simulink model "Nonelinear_Control_Project"  (R2018b)
settings: Solver=VariableStepAuto  StartTime=0.0  StopTime=80  FixedStep=0.01  RelTol=1e-3
InitFcn:
  | Initial_Data
StopFcn:
  | Plots
values from neighbouring files (symbols this model uses):
  alpha1 = 10    [Initial_Data.m]
  alpha2 = 10    [Initial_Data.m]
  alpha3 = 10    [Initial_Data.m]
  alpha4 = 10    [Initial_Data.m]
  b = 5    [Initial_Data.m]
  beta1 = 1    [Initial_Data.m]
  beta2 = 1    [Initial_Data.m]
  beta3 = 1    [Initial_Data.m]
  beta4 = 1    [Initial_Data.m]
  c3 = 1    [Initial_Data.m]
  c4 = 6    [Initial_Data.m]
  c7 = 1    [Initial_Data.m]
  c8 = 6    [Initial_Data.m]
  cpsi = 1    [Initial_Data.m]
  cz = 1    [Initial_Data.m]
  eta1 = 2    [Initial_Data.m]
  eta2 = 2    [Initial_Data.m]
  g = 9.81    [Initial_Data.m]
  Ix = 0.022    [Initial_Data.m]
  Iy = 0.022    [Initial_Data.m]
  Iz = 0.042    [Initial_Data.m]
  Jr = 0    [Initial_Data.m]
  k1 = 0.001    [Initial_Data.m]
  k2 = 0.001    [Initial_Data.m]
  k3 = 0.001    [Initial_Data.m]
  k4 = 0.0012    [Initial_Data.m]
  k5 = 0.0012    [Initial_Data.m]
  k6 = 0.0012    [Initial_Data.m]
  l = 0.21    [Initial_Data.m]
  m = 1.1    [Initial_Data.m]
  m1 = 1    [Initial_Data.m]
  m2 = 1    [Initial_Data.m]
  mperim1 = 7    [Initial_Data.m]
  mperim2 = 7    [Initial_Data.m]
  mperim3 = 7    [Initial_Data.m]
  mperim4 = 7    [Initial_Data.m]
  n1 = 3    [Initial_Data.m]
  n2 = 3    [Initial_Data.m]
  nperim1 = 9    [Initial_Data.m]
  nperim2 = 9    [Initial_Data.m]
  nperim3 = 9    [Initial_Data.m]
  nperim4 = 9    [Initial_Data.m]
  omega = 2000    [Initial_Data.m]
  Phi_desired = 0    [Initial_Data.m]
  Phi_dot_desired = 0    [Initial_Data.m]
  Phi_doubledot_desired = 0    [Initial_Data.m]
  Psi_desired = 0.5    [Initial_Data.m]
  Psi_dot_desired = 0    [Initial_Data.m]
  Psi_doubledot_desired = 0    [Initial_Data.m]
  Psi_tiersdot_desired = 0    [Initial_Data.m]
  Teta_desired = 0    [Initial_Data.m]
  Teta_dot_desired = 0    [Initial_Data.m]
  Teta_doubledot_desired = 0    [Initial_Data.m]
  x_desired = 0.6    [Initial_Data.m]
  x_dot_desired = 0    [Initial_Data.m]
  x_doubledot_desired = 0    [Initial_Data.m]
  x_tiersdot_desired = 0    [Initial_Data.m]
  y_desired = 0.6    [Initial_Data.m]
  y_dot_desired = 0    [Initial_Data.m]
  y_doubledot_desired = 0    [Initial_Data.m]
  y_tiersdot_desired = 0    [Initial_Data.m]
  z_desired = 0.6    [Initial_Data.m]
  z_dot_desired = 0    [Initial_Data.m]
  z_doubledot_desired = 0    [Initial_Data.m]
  z_tiersdot_desired = 0    [Initial_Data.m]
undefined symbols (not defined in the file or in its folder): c, CD0, CDalpha, CDalphadot, CDdelE, CDiH, CDq, CDu, CL0, CLalpha, CLalphadot, Clbeta, Clbetadot, CldelA, CLdelE, CldelR, CLiH, Clp, CLq, Clr, ClT, CLu, Cm0, Cmalpha, Cmalphadot, CmdelE, cmiH, Cmq, CmT1, CmTalpha, CmTu, Cmu, Cnbeta, Cnbetadot, CndelA, CndelR, Cnp, Cnr, CnTbeta, CTxu, CTy, CTz, Cybeta, Cybetadot, CydelA, CydelR, Cyp, Cyr, delE, iH, Ixx, Ixz, Iyy, Izz, Kp, mass, Ro, S, T1, taw ... (+3)
libraries: simulink x1
(part 1 of 2)
settings Model: Creator=Mehdi RJ  LastModifiedBy=User
settings DataIOCC: LimitDataPoints=on  SaveFormat=Array  SignalLoggingSaveFormat=ModelDataLogs
settings OptimizationCC: BlockReduction=off  BooleanDataType=off  LifeSpan=inf
settings DebuggingCC: SaveWithParameterizedLinksMsg=none  UnderspecifiedInitializationDetection=Classic  MergeDetectMultiDrivingBlocksExec=none  SignalResolutionControl=TryResolveAllWithWarning  MultiTaskDSMMsg=warning  MultiTaskCondExecSysMsg=none  SFUnexpectedBacktrackingDiag=warning  SFNoUnconditionalDefaultTransitionDiag=warning  SFExecutionAtInitializationDiag=none
settings HardwareCC: ProdBitPerPointer=32  ProdBitPerSizeT=32  ProdBitPerPtrDiffT=32  ProdLargestAtomicFloat=None  ProdIntDivRoundTo=Undefined  ProdEndianess=Unspecified  ProdWordSize=32  ProdHWDeviceType=32-bit Generic  TargetUnknown=on
settings ModelReferenceCC: PropagateSignalLabelsOutOfModel=off
settings SFSimCC: SimUseLocalCustomCode=off
settings RTWCC: RTWUseLocalCustomCode=off
settings CodeAppCC: StateflowObjectComments=on
settings GRTTargetCC: TargetLangStandard=C89/C90 (ANSI)  GeneratePreprocessorConditionals=Disable all
settings ConfigComp: CovMetricSettings=dw  CovHtmlReporting=on  CovSaveCumulativeToWorkspaceVar=on  CovSaveSingleToWorkspaceVar=on  CovExternalEMLEnable=off

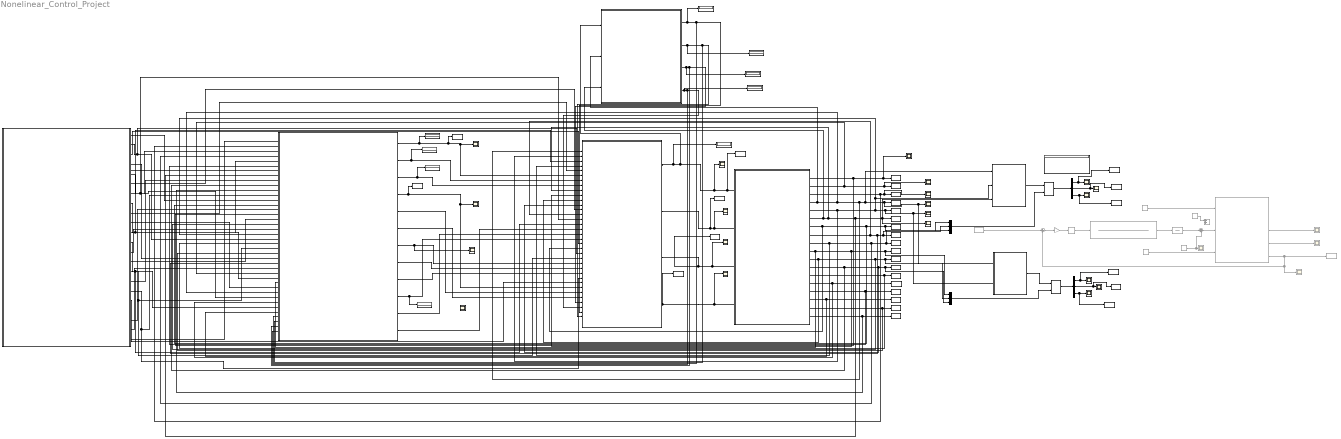
== system Nonelinear_Control_Project ==
  Add : Sum  Commented=on
  Airplane Dynamics : Subsystem  Commented=on
  "Controller " : Subsystem
  Demux : Demux  Outputs=3
  Demux2 : Demux  Outputs=3
  "Desired Values " : Subsystem
  Display{,1..9} (10 alike) : Display
  Gain1 : Gain  Commented=on  Gain=-1
  MATLAB Function : MATLAB Function  TreatAsAtomicUnit=on
  MATLAB Function1 : MATLAB Function  TreatAsAtomicUnit=on
  Matrix Multiply : Product  Multiplication=Matrix(*)
  Matrix Multiply1 : Product  Multiplication=Matrix(*)
  P : Scope
  PID Controller : simulink/Continuous/PID Controller  Commented=on  Controller=PID  Form=Parallel  TimeDomain=Continuous-time  SampleTime=-1  IntegratorMethod=Forward Euler  FilterMethod=Forward Euler  ControllerParametersSource=internal  P=9.72091586765638e-06  I=5.86209894111036e-08  D=9.64251086658951e-05  UseFilter=on  N=15.2377063472214  TunerSelectOption=Transfer Function Based (PID Tuner App)  InitialConditionSource=internal  InitialConditionForIntegrator=0  InitialConditionForFilter=0  DifferentiatorICPrevScaledInput=0  ExternalReset=none  TrackingMode=off  Kt=1  LimitOutput=off  UpperSaturationLimit=inf  LowerSaturationLimit=-inf  LinearizeAsGain=on  AntiWindupMode=none  Kb=1  POutMin=[]  POutMax=[]  IOutMin=[]  IOutMax=[]  DOutMin=[]  DOutMax=[]  NOutMin=[]  NOutMax=[]  SumOutMin=[]  SumOutMax=[]  SaturationOutMin=[]  SaturationOutMax=[]  PParamMin=[]  PParamMax=[]  IParamMin=[]  IParamMax=[]  DParamMin=[]  DParamMax=[]  NParamMin=[]  NParamMax=[]  KbParamMin=[]  KbParamMax=[]  KtParamMin=[]  KtParamMax=[]  KbOutMin=[]  KbOutMax=[]  KtOutMin=[]  KtOutMax=[]  IntegratorOutMin=[]  IntegratorOutMax=[]  FilterOutMin=[]  FilterOutMax=[]  SumI1OutMin=[]  SumI1OutMax=[]  SumI2OutMin=[]  SumI2OutMax=[]  SumI3OutMin=[]  SumI3OutMax=[]  SumI4OutMin=[]  SumI4OutMax=[]  SumDOutMin=[]  SumDOutMax=[]  DifferentiatorOutMin=[]  DifferentiatorOutMax=[]  FilterDiffOutCoefMin=[]  FilterDiffOutCoefMax=[]  ReciprocalOutMin=[]  ReciprocalOutMax=[]  SumDenOutMin=[]  SumDenOutMax=[]  SumNumOutMin=[]  SumNumOutMax=[]  DivideOutMin=[]  DivideOutMax=[]  IntegratorContinuousStateAttributes=''  IntegratorStateMustResolveToSignalObject=off  IntegratorRTWStateStorageClass=Auto  FilterContinuousStateAttributes=''  FilterStateMustResolveToSignalObject=off  FilterRTWStateStorageClass=Auto  ParallelPVariant=InternalParameters  IdealPVariant=Disabled  IVariant=InternalParameters  DVariant=InternalParameters  IntegratorVariant=Continuous  SatVariant=Disabled  AWVariant=Passthrough  PCopyVariant=Disabled  TRVariant=Disabled  FdbkBlocksVariant=Forward  IdealPFdbkVariant=Disabled  SatFdbkVariant=Disabled  DerivativeFilterVariant=ContFilter  NVariant=InternalParameters  NCopyVariant=Disabled  FilterICVariant=InternalICsFilter  IntegratorICVariant=InternalICs  ExternalResetVariant=Disabled  TRSumVariant=Passthrough  SumFdbkVariant=Disabled  SumVariant=Sum_PID
  Pilot Transfer Function : TransferFcn  Commented=on  Numerator=[(- Kp*TL* taw) (- Kp*taw+ 2*Kp*TL) (2*Kp)]  Denominator=[(TI*TN*taw) (TN*taw+TI*taw+2*TI*TN) (taw+2*TN+2*TI) 2]
  Pulse Generator : DiscretePulseGenerator  Commented=on  PulseType=Time based  Amplitude=0.0175*5  Period=2000  PhaseDelay=800
  Q : Scope
  Quadrotordynamics : Subsystem
  R : Scope
  Scope{,1..3} (4 alike) : Scope  Commented=on
  Scope{4..17} (14 alike) : Scope
  Subsystem : Subsystem
  Sum : Sum  Commented=on  Inputs=|+-
  Sum1 : Sum  Commented=on  Inputs=|++
  TSMC and SMC Manifolds : Subsystem
  To Workspace : ToWorkspace  VariableName=x  SaveFormat=Timeseries  SampleTime=-1
  To Workspace1 : ToWorkspace  VariableName=y  SaveFormat=Timeseries  SampleTime=-1
  To Workspace10 : ToWorkspace  VariableName=Tetadot  SaveFormat=Timeseries  SampleTime=-1
  To Workspace11 : ToWorkspace  VariableName=Psidot  SaveFormat=Timeseries  SampleTime=-1
  To Workspace12 : ToWorkspace  VariableName=xddot  SaveFormat=Timeseries  SampleTime=-1
  To Workspace13 : ToWorkspace  VariableName=yddot  SaveFormat=Timeseries  SampleTime=-1
  To Workspace14 : ToWorkspace  VariableName=zddot  SaveFormat=Timeseries  SampleTime=-1
  To Workspace15 : ToWorkspace  VariableName=Phiddot  SaveFormat=Timeseries  SampleTime=-1
  To Workspace16 : ToWorkspace  VariableName=Tetaddot  SaveFormat=Timeseries  SampleTime=-1
  To Workspace17 : ToWorkspace  VariableName=Psiddot  SaveFormat=Timeseries  SampleTime=-1
  To Workspace18 : ToWorkspace  VariableName=P  SaveFormat=Timeseries  SampleTime=-1
  To Workspace19 : ToWorkspace  VariableName=Q  SaveFormat=Timeseries  SampleTime=-1
  To Workspace2 : ToWorkspace  VariableName=z  SaveFormat=Timeseries  SampleTime=-1
  To Workspace20 : ToWorkspace  Commented=on  VariableName=h  SaveFormat=Timeseries  SampleTime=-1
  To Workspace21 : ToWorkspace  VariableName=R  SaveFormat=Timeseries  SampleTime=-1
  To Workspace22 : ToWorkspace  VariableName=U  SaveFormat=Timeseries  SampleTime=-1
  To Workspace23 : ToWorkspace  VariableName=V  SaveFormat=Timeseries  SampleTime=-1
  To Workspace24 : ToWorkspace  VariableName=W  SaveFormat=Timeseries  SampleTime=-1
  To Workspace25 : ToWorkspace  VariableName=u1  SaveFormat=Timeseries  SampleTime=-1
  To Workspace26 : ToWorkspace  VariableName=u2  SaveFormat=Timeseries  SampleTime=-1
  To Workspace27 : ToWorkspace  VariableName=u3  SaveFormat=Timeseries  SampleTime=-1
  To Workspace28 : ToWorkspace  VariableName=u4  SaveFormat=Timeseries  SampleTime=-1
  To Workspace29 : ToWorkspace  VariableName=s1  SaveFormat=Timeseries  SampleTime=-1
  To Workspace3 : ToWorkspace  VariableName=Phi  SaveFormat=Timeseries  SampleTime=-1
  To Workspace30 : ToWorkspace  VariableName=s3  SaveFormat=Timeseries  SampleTime=-1
  To Workspace4 : ToWorkspace  VariableName=Teta  SaveFormat=Timeseries  SampleTime=-1
  To Workspace5 : ToWorkspace  VariableName=Psi  SaveFormat=Timeseries  SampleTime=-1
  To Workspace6 : ToWorkspace  VariableName=xdot  SaveFormat=Timeseries  SampleTime=-1
  To Workspace7 : ToWorkspace  VariableName=ydot  SaveFormat=Timeseries  SampleTime=-1
  To Workspace8 : ToWorkspace  VariableName=zdot  SaveFormat=Timeseries  SampleTime=-1
  To Workspace9 : ToWorkspace  VariableName=Phidot  SaveFormat=Timeseries  SampleTime=-1
  Transfer Fcn1 : TransferFcn  Commented=on  Numerator=[10]  Denominator=[1 10]
  U : Scope
  V : Scope
  Vector Concatenate : Concatenate  NumInputs=3
  Vector Concatenate1 : Concatenate  NumInputs=3
  W : Scope
  delA : Constant  Commented=on  Value=0
  delA1 : Constant  Commented=on  Value=delE
  delR : Constant  Commented=on  Value=0
  h : Constant  Commented=on  Value=20000
  wires:
  delR/1 -> Airplane Dynamics/3(delR)
  delA/1 -> Airplane Dynamics/1(delA)
  Airplane Dynamics/3(Theta) -> Scope/1
  h/1 -> Sum/1
  Airplane Dynamics/4(Q) -> Scope1/1
  Pulse Generator/1 -> Sum1/2, Scope2/1
  Sum/1 -> Gain1/1
  Gain1/1 -> PID Controller/1
  Airplane Dynamics/5(h) -> Sum/2, Scope3/1, To Workspace20/1
  Pilot Transfer Function/1 -> Transfer Fcn1/1
  Transfer Fcn1/1 -> Sum1/1
  PID Controller/1 -> Pilot Transfer Function/1
  delA1/1 -> Add/1
  Sum1/1 -> Airplane Dynamics/2(delE)
  Quadrotordynamics/1(x) -> TSMC and SMC Manifolds/16(x), Scope4/1, To Workspace/1
  Quadrotordynamics/2(y) -> TSMC and SMC Manifolds/28(y), Scope5/1, To Workspace1/1
  Quadrotordynamics/3(z) -> TSMC and SMC Manifolds/2(z), Scope6/1, To Workspace2/1
  Quadrotordynamics/4(Phi) -> Subsystem/2(Phi), TSMC and SMC Manifolds/32(Phi), To Workspace3/1, MATLAB Function1/1(Phi), Scope7/1, MATLAB Function/1(Phi), "Controller "/1(Phi)
  "Controller "/1(u1) -> Display7/1, Subsystem/1(u1), Scope10/1, To Workspace25/1, Quadrotordynamics/1(u1)
  "Controller "/2(u2) -> To Workspace26/1, Scope11/1, Quadrotordynamics/2(u2)
  "Controller "/3(u3) -> Scope12/1, Quadrotordynamics/3(u3), To Workspace27/1
  "Controller "/4(u4) -> Scope13/1, Quadrotordynamics/4(u4), To Workspace28/1
  Quadrotordynamics/7(xdot) -> "Controller "/21(xdot), TSMC and SMC Manifolds/14(xdot), Vector Concatenate/1, To Workspace6/1
  Quadrotordynamics/5(Teta) -> "Controller "/2(Teta), TSMC and SMC Manifolds/20(Teta), MATLAB Function/2(Teta), MATLAB Function1/2(Teta), Scope8/1, To Workspace4/1
  Quadrotordynamics/10(Phidot) -> TSMC and SMC Manifolds/30(Phidot), "Controller "/10(Phidot), Vector Concatenate1/1, To Workspace9/1
  Quadrotordynamics/11(Tetadot) -> "Controller "/11(Tetadot), TSMC and SMC Manifolds/18(Tetadot), Vector Concatenate1/2, To Workspace10/1
  Quadrotordynamics/8(ydot) -> "Controller "/14(ydot), TSMC and SMC Manifolds/26(ydot), Vector Concatenate/2, To Workspace7/1
  TSMC and SMC Manifolds/1("s1 ") -> Display/1, To Workspace29/1, "Controller "/6(s1), Scope14/1
  TSMC and SMC Manifolds/2("s1dot ") -> Display8/1, "Controller "/7(s1dot)
  TSMC and SMC Manifolds/3("s2 ") -> Display1/1, "Controller "/8(s2)
  TSMC and SMC Manifolds/4("s3 ") -> To Workspace30/1, Scope15/1, "Controller "/29(s3)
  TSMC and SMC Manifolds/5("s3dot ") -> "Controller "/30(s3dot)
  TSMC and SMC Manifolds/6("s4 ") -> "Controller "/31(s4)
  TSMC and SMC Manifolds/7("s5 ") -> Scope16/1, "Controller "/24(s5)
  TSMC and SMC Manifolds/8("s5dot  ") -> "Controller "/25(s5dot)
  TSMC and SMC Manifolds/9("s6 ") -> "Controller "/26(s6)
  TSMC and SMC Manifolds/10("s7 ") -> Display2/1, "Controller "/19(s7)
  TSMC and SMC Manifolds/11("s7dot ") -> "Controller "/18(s7dot)
  TSMC and SMC Manifolds/12("s8 ") -> "Controller "/17(s8)
  Quadrotordynamics/6(Psi) -> Subsystem/3(Psi), Scope9/1, To Workspace5/1, MATLAB Function/3(Psi), TSMC and SMC Manifolds/8(Psi), "Controller "/9(Psi)
  Quadrotordynamics/12(Psidot) -> "Controller "/12(Psidot), Vector Concatenate1/3, To Workspace11/1, TSMC and SMC Manifolds/10(Psidot)
  Quadrotordynamics/15(zddot) -> TSMC and SMC Manifolds/6(zdoubledot), To Workspace14/1
  Quadrotordynamics/13(xddot) -> TSMC and SMC Manifolds/22(xdoubledot), To Workspace12/1
  Quadrotordynamics/14(yddot) -> TSMC and SMC Manifolds/34(ydoubledot), To Workspace13/1
  Quadrotordynamics/17(Tetaddot) -> TSMC and SMC Manifolds/24(Tetadoubledot), To Workspace16/1
  Quadrotordynamics/18(Psiddot) -> TSMC and SMC Manifolds/11(Psidoubledot), To Workspace17/1
  Quadrotordynamics/16(Phiddot) -> To Workspace15/1, TSMC and SMC Manifolds/36(Phidoubledot)
  "Desired Values "/7("z_dot_desired ") -> TSMC and SMC Manifolds/3(z_dot_desired)
  "Desired Values "/16("Psi_dot_desired ") -> TSMC and SMC Manifolds/9(Psi_dot_desired)
  "Desired Values "/17("Psi_doubledot_desired ") -> "Controller "/27(Psi_doubledot_desired), TSMC and SMC Manifolds/12(Psi_doubledot_desired)
  "Desired Values "/1("x_dot_desired ") -> TSMC and SMC Manifolds/13(x_dot_desired)
  "Desired Values "/2("x_doubledot_desired ") -> "Controller "/22(x_doubledot_desired), TSMC and SMC Manifolds/21(x_doubledot_desired)
  "Desired Values "/4("y_dot_desired ") -> TSMC and SMC Manifolds/25(y_dot_desired)
  "Desired Values "/5("y_doubledot_desired ") -> "Controller "/15(y_doubledot_desired), TSMC and SMC Manifolds/33(y_doubledot_desired)
  "Desired Values "/10("Phi_desired ") -> TSMC and SMC Manifolds/31(Phi_desired)
  "Desired Values "/11("Phi_dot_desired ") -> TSMC and SMC Manifolds/29(Phi_dot_desired)
  "Desired Values "/12("Phi_doubledot_desired ") -> "Controller "/16(Phi_doubledot_desired), TSMC and SMC Manifolds/35(Phi_doubledot_desired)
  "Desired Values "/13("Teta_desired ") -> TSMC and SMC Manifolds/19(Teta_desired)
  "Desired Values "/14("Teta_dot_desired  ") -> TSMC and SMC Manifolds/17(Teta_dot_desired)
  "Desired Values "/15("Teta_doubledot_desired ") -> "Controller "/23(Teta_doubledot_desired), TSMC and SMC Manifolds/23(Teta_doubledot_desired)
  "Desired Values "/8("z_doubledot_desired ") -> "Controller "/3(z_doubledot_desired), TSMC and SMC Manifolds/5(z_doubledot_desired)
  "Desired Values "/9("z_tiersdot_desired ") -> "Controller "/5(z_tiersdot_desired)
  "Desired Values "/6("y_tiersdot_desired ") -> "Controller "/13(y_tiersdot_desired)
  "Desired Values "/3("x_tiersdot_desired ") -> "Controller "/20(x_tiersdot_desired)
  "Desired Values "/18("Psi_tiersdot_desired ") -> "Controller "/28(Psi_tiersdot_desired)
  Subsystem/1("c1 ") -> Display3/1, TSMC and SMC Manifolds/37(c1), "Controller "/34(c1)
  Subsystem/3("c5 ") -> Display5/1, TSMC and SMC Manifolds/39(c5), "Controller "/32(c5)
  Subsystem/4("c6 ") -> Display6/1, TSMC and SMC Manifolds/40(c6), "Controller "/33(c6)
  Subsystem/2("c2 ") -> Display4/1, TSMC and SMC Manifolds/38(c2), "Controller "/35(c2)
  MATLAB Function/1(DCM) -> Matrix Multiply/1
  Quadrotordynamics/9(zdot) -> "Controller "/4(zdot), TSMC and SMC Manifolds/4("zdot "), Vector Concatenate/3, To Workspace8/1
  Vector Concatenate/1 -> Matrix Multiply/2
  Matrix Multiply/1 -> Demux/1
  Demux/3 -> To Workspace24/1, W/1
  Demux/2 -> To Workspace23/1, V/1
  Demux/1 -> To Workspace22/1, U/1
  MATLAB Function1/1(DCM) -> Matrix Multiply1/1
  Vector Concatenate1/1 -> Matrix Multiply1/2
  Demux2/1 -> To Workspace18/1, P/1
  Demux2/2 -> To Workspace19/1, Q/1
  Demux2/3 -> To Workspace21/1, R/1
  Matrix Multiply1/1 -> Demux2/1
  "Desired Values "/19("Psi_desired ") -> TSMC and SMC Manifolds/7("Psi_desired ")
  "Desired Values "/20("x_desired ") -> TSMC and SMC Manifolds/15(x_desired)
  "Desired Values "/21("y_desired ") -> TSMC and SMC Manifolds/27(y_desired)
  "Desired Values "/22("z_desired ") -> TSMC and SMC Manifolds/1("z_desired ")

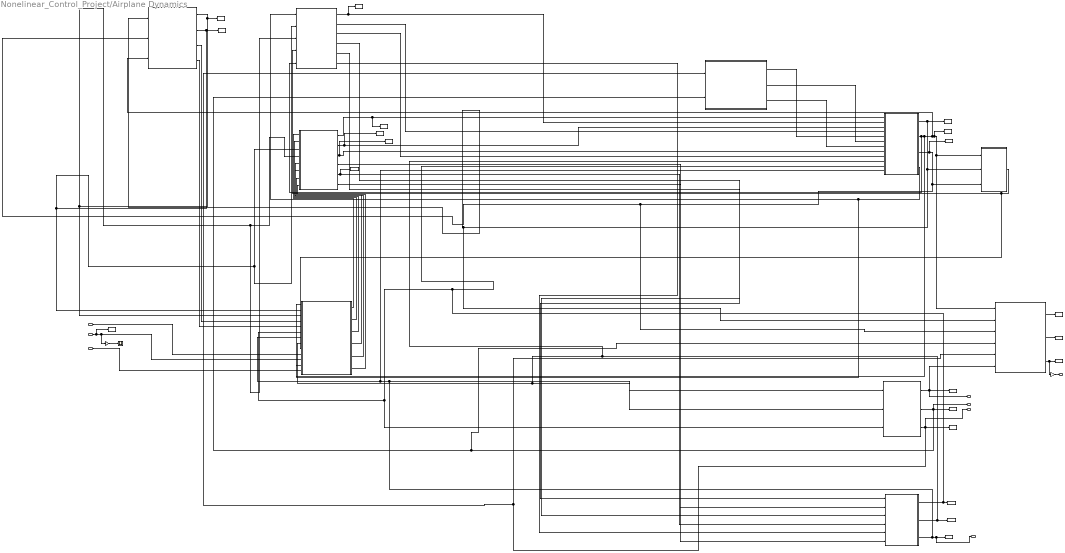
== system Nonelinear_Control_Project/Airplane Dynamics ==
  delA : Inport
  delE : Inport  Port=2
  delR : Inport  Port=3
  AnglesBlock : Subsystem
  Angular Velocities (P,Q,R) : Subsystem
  Body Aerodynamic Forces and Moments (FAxB,FAyB,FAzB,LAB,MAB,NAB) : Subsystem
  Dynamic Pressure : Subsystem
  Euler's Angles (Phi,Theta,Psi) : Subsystem
  GBlock : Subsystem
  Gain : Gain  Gain=-1
  Gain1 : Gain  Gain=180/pi
  Linear Velocities (U,V,W) : Subsystem
  Navigation : Subsystem
  Scope : Scope
  Stability Aerodunamic Forces and Moments (FAxS,FAyS,FAzS,LAS,MAS,NAS) : Subsystem
  Thrust Forces and Moments (FTx,FTy,FTz,LT,MT,NT) : Subsystem
  To Workspace : ToWorkspace  VariableName=XInertia  SaveFormat=Timeseries  SampleTime=-1
  To Workspace1 : ToWorkspace  VariableName=YInertia  SaveFormat=Timeseries  SampleTime=-1
  To Workspace10 : ToWorkspace  VariableName=Q  SaveFormat=Timeseries  SampleTime=-1
  To Workspace11 : ToWorkspace  VariableName=R  SaveFormat=Timeseries  SampleTime=-1
  To Workspace12 : ToWorkspace  VariableName=P  SaveFormat=Timeseries  SampleTime=-1
  To Workspace13 : ToWorkspace  VariableName=W  SaveFormat=Timeseries  SampleTime=-1
  To Workspace14 : ToWorkspace  VariableName=FAzB  SaveFormat=Timeseries  SampleTime=-1
  To Workspace15 : ToWorkspace  VariableName=FTx  SaveFormat=Timeseries  SampleTime=-1
  To Workspace16 : ToWorkspace  VariableName=FAxB  SaveFormat=Timeseries  SampleTime=-1
  To Workspace17 : ToWorkspace  VariableName=FAyB  SaveFormat=Timeseries  SampleTime=-1
  To Workspace18 : ToWorkspace  VariableName=V  SaveFormat=Timeseries  SampleTime=-1
  To Workspace19 : ToWorkspace  VariableName=delE  SaveFormat=Timeseries  SampleTime=-1
  To Workspace2 : ToWorkspace  VariableName=ZInertia  SaveFormat=Timeseries  SampleTime=-1
  To Workspace3 : ToWorkspace  VariableName=alpha  SaveFormat=Timeseries  SampleTime=-1
  To Workspace4 : ToWorkspace  VariableName=beta  SaveFormat=Timeseries  SampleTime=-1
  To Workspace5 : ToWorkspace  VariableName=U  SaveFormat=Timeseries  SampleTime=-1
  To Workspace6 : ToWorkspace  VariableName=Psi  SaveFormat=Timeseries  SampleTime=-1
  To Workspace7 : ToWorkspace  VariableName=Phi  SaveFormat=Timeseries  SampleTime=-1
  To Workspace8 : ToWorkspace  VariableName=Theta  SaveFormat=Timeseries  SampleTime=-1
  To Workspace9 : ToWorkspace  VariableName=MAB  SaveFormat=Timeseries  SampleTime=-1
  Psi : Outport
  Phi : Outport  Port=2
  Theta : Outport  Port=3
  Q : Outport  Port=4
  h : Outport  Port=5
  wires:
  AnglesBlock/2(alpha) -> To Workspace3/1, Thrust Forces and Moments (FTx,FTy,FTz,LT,MT,NT)/2(alpha), Body Aerodynamic Forces and Moments (FAxB,FAyB,FAzB,LAB,MAB,NAB)/3(alpha), Stability Aerodunamic Forces and Moments (FAxS,FAyS,FAzS,LAS,MAS,NAS)/2(alpha)
  Stability Aerodunamic Forces and Moments (FAxS,FAyS,FAzS,LAS,MAS,NAS)/1(FAxS) -> Body Aerodynamic Forces and Moments (FAxB,FAyB,FAzB,LAB,MAB,NAB)/1(FAxS)
  Thrust Forces and Moments (FTx,FTy,FTz,LT,MT,NT)/2(FTy) -> Linear Velocities (U,V,W)/4(FTy)
  Thrust Forces and Moments (FTx,FTy,FTz,LT,MT,NT)/5(MT) -> Angular Velocities (P,Q,R)/3(MT)
  Angular Velocities (P,Q,R)/1(P) -> To Workspace12/1, Linear Velocities (U,V,W)/11(P), Stability Aerodunamic Forces and Moments (FAxS,FAyS,FAzS,LAS,MAS,NAS)/6(P), Euler's Angles (Phi,Theta,Psi)/3(P)
  AnglesBlock/3(betadot) -> Stability Aerodunamic Forces and Moments (FAxS,FAyS,FAzS,LAS,MAS,NAS)/4("betadot ")
  Euler's Angles (Phi,Theta,Psi)/1(Psi) -> To Workspace6/1, Navigation/6(Psi), Psi/1
  delR/1 -> Stability Aerodunamic Forces and Moments (FAxS,FAyS,FAzS,LAS,MAS,NAS)/13(delR)
  Body Aerodynamic Forces and Moments (FAxB,FAyB,FAzB,LAB,MAB,NAB)/4(LAB) -> Angular Velocities (P,Q,R)/2(LAB)
  Body Aerodynamic Forces and Moments (FAxB,FAyB,FAzB,LAB,MAB,NAB)/5(MAB) -> To Workspace9/1, Angular Velocities (P,Q,R)/4(MAB)
  Linear Velocities (U,V,W)/3(W) -> To Workspace13/1, Dynamic Pressure/3(W), AnglesBlock/2(W), Navigation/3(W)
  Angular Velocities (P,Q,R)/3(Q) -> Euler's Angles (Phi,Theta,Psi)/2(Q), Linear Velocities (U,V,W)/12(Q), Stability Aerodunamic Forces and Moments (FAxS,FAyS,FAzS,LAS,MAS,NAS)/7(Q), Q/1, To Workspace10/1
  Linear Velocities (U,V,W)/1(V) -> To Workspace18/1, Dynamic Pressure/2(V), AnglesBlock/1(V), Navigation/2(V)
  Euler's Angles (Phi,Theta,Psi)/3(Theta) -> To Workspace8/1, GBlock/1(Theta), Navigation/5(Theta), Theta/1
  AnglesBlock/1("beta ") -> To Workspace4/1, Body Aerodynamic Forces and Moments (FAxB,FAyB,FAzB,LAB,MAB,NAB)/4(beta), Thrust Forces and Moments (FTx,FTy,FTz,LT,MT,NT)/3(beta), Stability Aerodunamic Forces and Moments (FAxS,FAyS,FAzS,LAS,MAS,NAS)/3(beta)
  Linear Velocities (U,V,W)/4(delU) -> Stability Aerodunamic Forces and Moments (FAxS,FAyS,FAzS,LAS,MAS,NAS)/1(delU), Thrust Forces and Moments (FTx,FTy,FTz,LT,MT,NT)/1(delU)
  Thrust Forces and Moments (FTx,FTy,FTz,LT,MT,NT)/3(FTz) -> Linear Velocities (U,V,W)/9(FTz)
  Navigation/2(YInertia) -> To Workspace1/1
  Stability Aerodunamic Forces and Moments (FAxS,FAyS,FAzS,LAS,MAS,NAS)/4(LAS) -> Body Aerodynamic Forces and Moments (FAxB,FAyB,FAzB,LAB,MAB,NAB)/6(LAS)
  Euler's Angles (Phi,Theta,Psi)/2(Phi) -> To Workspace7/1, Navigation/4(Phi), GBlock/2("Phi "), Phi/1
  Body Aerodynamic Forces and Moments (FAxB,FAyB,FAzB,LAB,MAB,NAB)/3(FAzB) -> To Workspace14/1, Linear Velocities (U,V,W)/8(FAzB)
  Stability Aerodunamic Forces and Moments (FAxS,FAyS,FAzS,LAS,MAS,NAS)/2(FAyS) -> Body Aerodynamic Forces and Moments (FAxB,FAyB,FAzB,LAB,MAB,NAB)/2(FAyS)
  GBlock/2(gy) -> Linear Velocities (U,V,W)/6(gy)
  AnglesBlock/4(alphadot) -> Stability Aerodunamic Forces and Moments (FAxS,FAyS,FAzS,LAS,MAS,NAS)/5(alphadot)
  Navigation/1(XInertia) -> To Workspace/1
  Thrust Forces and Moments (FTx,FTy,FTz,LT,MT,NT)/1(FTx) -> To Workspace15/1, Linear Velocities (U,V,W)/2(FTx)
  Stability Aerodunamic Forces and Moments (FAxS,FAyS,FAzS,LAS,MAS,NAS)/5(MAS) -> Body Aerodynamic Forces and Moments (FAxB,FAyB,FAzB,LAB,MAB,NAB)/7(MAS)
  Thrust Forces and Moments (FTx,FTy,FTz,LT,MT,NT)/6(NT) -> Angular Velocities (P,Q,R)/5(NT)
  Stability Aerodunamic Forces and Moments (FAxS,FAyS,FAzS,LAS,MAS,NAS)/6(NAS) -> Body Aerodynamic Forces and Moments (FAxB,FAyB,FAzB,LAB,MAB,NAB)/8(NAS)
  Navigation/3(ZInertia) -> Gain/1, To Workspace2/1
  Linear Velocities (U,V,W)/2(U) -> Thrust Forces and Moments (FTx,FTy,FTz,LT,MT,NT)/5(U), Stability Aerodunamic Forces and Moments (FAxS,FAyS,FAzS,LAS,MAS,NAS)/12(U), AnglesBlock/3(U), To Workspace5/1, Navigation/1(U), Dynamic Pressure/1(U)
  Stability Aerodunamic Forces and Moments (FAxS,FAyS,FAzS,LAS,MAS,NAS)/3(FAzS) -> Body Aerodynamic Forces and Moments (FAxB,FAyB,FAzB,LAB,MAB,NAB)/5(FAzS)
  Dynamic Pressure/1(q1) -> Stability Aerodunamic Forces and Moments (FAxS,FAyS,FAzS,LAS,MAS,NAS)/9(q1), Thrust Forces and Moments (FTx,FTy,FTz,LT,MT,NT)/4(q1)
  Body Aerodynamic Forces and Moments (FAxB,FAyB,FAzB,LAB,MAB,NAB)/6(NAB) -> Angular Velocities (P,Q,R)/6(NAB)
  GBlock/1(gx) -> Linear Velocities (U,V,W)/5(gx)
  GBlock/3(gz) -> Linear Velocities (U,V,W)/7(gz)
  Body Aerodynamic Forces and Moments (FAxB,FAyB,FAzB,LAB,MAB,NAB)/1(FAxB) -> To Workspace16/1, Linear Velocities (U,V,W)/1(FAxB)
  Angular Velocities (P,Q,R)/2(R) -> To Workspace11/1, Stability Aerodunamic Forces and Moments (FAxS,FAyS,FAzS,LAS,MAS,NAS)/8(R), Euler's Angles (Phi,Theta,Psi)/1(R), Linear Velocities (U,V,W)/10(R)
  Thrust Forces and Moments (FTx,FTy,FTz,LT,MT,NT)/4(LT) -> Angular Velocities (P,Q,R)/1(LT)
  Body Aerodynamic Forces and Moments (FAxB,FAyB,FAzB,LAB,MAB,NAB)/2(FAyB) -> To Workspace17/1, Linear Velocities (U,V,W)/3(FAyB)
  delA/1 -> Stability Aerodunamic Forces and Moments (FAxS,FAyS,FAzS,LAS,MAS,NAS)/10(delA)
  Gain/1 -> h/1
  delE/1 -> To Workspace19/1, Gain1/1, Stability Aerodunamic Forces and Moments (FAxS,FAyS,FAzS,LAS,MAS,NAS)/11(delE)
  Gain1/1 -> Scope/1

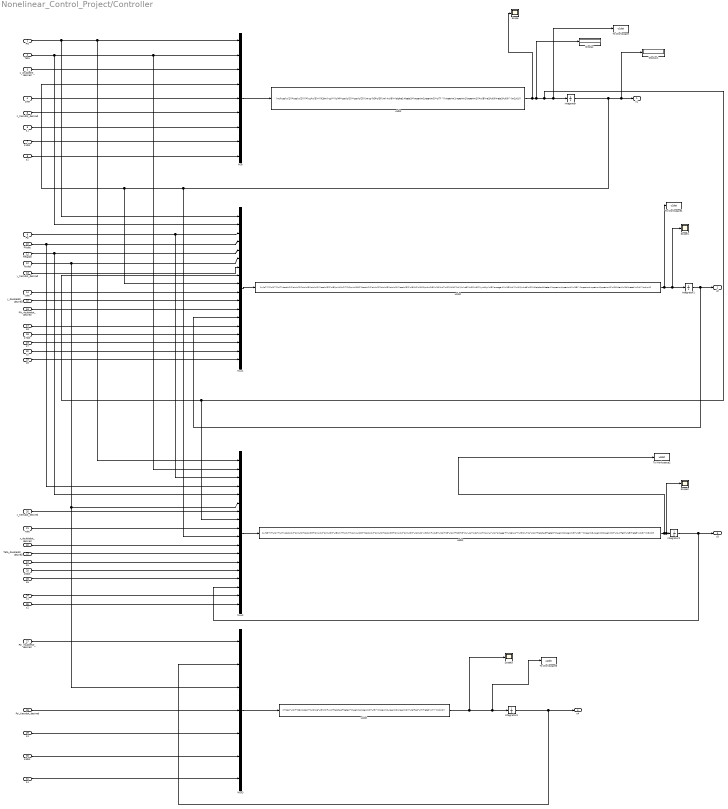
== system Nonelinear_Control_Project/Controller  ==
  Phi : Inport
  Teta : Inport  Port=2
  z_doubledot_desired : Inport  Port=3
  zdot : Inport  Port=4
  z_tiersdot_desired : Inport  Port=5
  s1 : Inport  Port=6
  s1dot : Inport  Port=7
  s2 : Inport  Port=8
  Psi : Inport  Port=9
  Phidot : Inport  Port=10
  Tetadot : Inport  Port=11
  Psidot : Inport  Port=12
  y_tiersdot_desired : Inport  Port=13
  ydot : Inport  Port=14
  y_doubledot_desired : Inport  Port=15
  Phi_doubledot_desired : Inport  Port=16
  s8 : Inport  Port=17
  s7dot : Inport  Port=18
  s7 : Inport  Port=19
  x_tiersdot_desired : Inport  Port=20
  xdot : Inport  Port=21
  x_doubledot_desired : Inport  Port=22
  Teta_doubledot_desired : Inport  Port=23
  s5 : Inport  Port=24
  s5dot : Inport  Port=25
  s6 : Inport  Port=26
  Psi_doubledot_desired : Inport  Port=27
  Psi_tiersdot_desired : Inport  Port=28
  s3 : Inport  Port=29
  s3dot : Inport  Port=30
  s4 : Inport  Port=31
  c5 : Inport  Port=32
  c6 : Inport  Port=33
  c1 : Inport  Port=34
  c2 : Inport  Port=35
  Display : Display
  Display1 : Display
  Integrator : Integrator  InitialCondition=0.0000001
  Integrator1 : Integrator
  Integrator2 : Integrator
  Integrator3 : Integrator
  Mux : Mux  Inputs=9
  Mux1 : Mux  Inputs=18
  Mux2 : Mux  Inputs=18
  Mux3 : Mux  Inputs=7
  Scope{,1..3} (4 alike) : Scope
  To Workspace : ToWorkspace  VariableName=u1dot  SaveFormat=Timeseries  SampleTime=-1
  To Workspace1 : ToWorkspace  VariableName=u2dot  SaveFormat=Timeseries  SampleTime=-1
  To Workspace2 : ToWorkspace  VariableName=u3dot  SaveFormat=Timeseries  SampleTime=-1
  To Workspace3 : ToWorkspace  VariableName=u4dot  SaveFormat=Timeseries  SampleTime=-1
  u1dot : Fcn  Expr=(m/(cos(u(1))*cos(u(2))))*(cz*u(3)+((k3/m)-cz)*((u(4)*cos(u(1))*cos(u(2)))/m-g-(k3*u(5))/m)+u(6)+(alpha1+beta1*(mperim1/nperim1)*u(7)^((mperim1-nperim1)/nperim1))*u(8)+e1*u(9)+eta1*u(9)^(m1/n1))
  u2dot : Fcn  Expr=(Ix/(c7*l))*(u(17)*(u(7)-(cos(u(1))*sin(u(2))*sin(u(3))-sin(u(1))*cos(u(3)))*u(8)/m)+((u(17)*k2/m)-u(18))*((cos(u(1))*sin(u(2))*sin(u(3))-sin(u(1))*cos(u(3)))*u(9)-k2*u(10))/m+u(18)*u(11)+c7*u(12)+((c7*k4*l/Ix)-c8)*(u(5)*u(6)*(Iy-Iz)+Jr*u(5)*omega+l*u(13)-k4*l*u(4))/Ix+c8*u(12)+(alpha4+beta4*(mperim4/nperim4)*u(16)^((mperim4-nperim4)/nperim4))*u(15)+e4*u(14)+eta4*u(14)^(m4/n4))
  u3dot : Fcn  Expr=(Iy/(c3*l))*(u(17)*(u(7)-(cos(u(1))*sin(u(2))*cos(u(3))+sin(u(1))*sin(u(3)))*u(8)/m)+((u(17)*k1/m)-u(18))*((cos(u(1))*sin(u(2))*cos(u(3))+sin(u(1))*sin(u(3)))*u(10)-k1*u(9))/m+u(18)*u(11)+c3*u(12)+((c3*k5*l/Iy)-c4)*(u(6)*u(4)*(Iz-Ix)-Jr*u(4)*omega+l*u(16)-k4*l*u(5))/Iy+c4*u(12)+(alpha3+beta3*(mperim3/nperim3)*u(13)^((mperim3-nperim3)/nperim3))*u(14)+e3*u(15)+eta3*u(15)^(m3/n3))
  u4dot : Fcn  Expr=Iz*(cpsi*u(1)+((k6/Iz)-cpsi)*((u(2)-k6*u(3))/Iz)+u(4)+(alpha2+beta2*(mperim2/nperim2)*u(5)^((mperim2-nperim2)/nperim2))*u(6)+e2*u(7)+eta2*u(7)^(m2/n2))
  u1 : Outport
  u2 : Outport  Port=2
  u3 : Outport  Port=3
  u4 : Outport  Port=4
  wires:
  z_doubledot_desired/1 -> Mux/3
  u1dot/1 -> Scope/1, Display/1, Mux2/8, Mux1/8, To Workspace/1, Integrator/1
  zdot/1 -> Mux/5
  z_tiersdot_desired/1 -> Mux/6
  s1/1 -> Mux/7
  s1dot/1 -> Mux/8
  s2/1 -> Mux/9
  Mux1/1 -> u2dot/1
  u2dot/1 -> To Workspace1/1, Scope1/1, Integrator1/1
  Psi/1 -> Mux2/3, Mux1/3
  Phidot/1 -> Mux2/4, Mux1/4
  Tetadot/1 -> Mux2/5, Mux1/5
  y_tiersdot_desired/1 -> Mux1/7
  ydot/1 -> Mux1/10
  y_doubledot_desired/1 -> Mux1/11
  Phi_doubledot_desired/1 -> Mux1/12
  s8/1 -> Mux1/14
  s7dot/1 -> Mux1/15
  s7/1 -> Mux1/16
  Integrator2/1 -> u3/1, Mux2/16
  u3dot/1 -> To Workspace2/1, Scope2/1, Integrator2/1
  Mux2/1 -> u3dot/1
  Phi/1 -> Mux2/1, Mux/1, Mux1/1
  Teta/1 -> Mux2/2, Mux/2, Mux1/2
  x_tiersdot_desired/1 -> Mux2/7
  xdot/1 -> Mux2/9
  Integrator/1 -> Mux2/10, Mux1/9, Mux/4, Display1/1, u1/1
  x_doubledot_desired/1 -> Mux2/11
  Teta_doubledot_desired/1 -> Mux2/12
  s5/1 -> Mux2/13
  s5dot/1 -> Mux2/14
  s6/1 -> Mux2/15
  Mux3/1 -> u4dot/1
  u4dot/1 -> Scope3/1, To Workspace3/1, Integrator3/1
  Integrator3/1 -> u4/1, Mux3/2
  Psi_doubledot_desired/1 -> Mux3/1
  Psidot/1 -> Mux3/3, Mux2/6, Mux1/6
  Psi_tiersdot_desired/1 -> Mux3/4
  s4/1 -> Mux3/7
  s3/1 -> Mux3/5
  s3dot/1 -> Mux3/6
  Integrator1/1 -> Mux1/13, u2/1
  c5/1 -> Mux1/17
  c6/1 -> Mux1/18
  c1/1 -> Mux2/17
  c2/1 -> Mux2/18
  Mux/1 -> u1dot/1

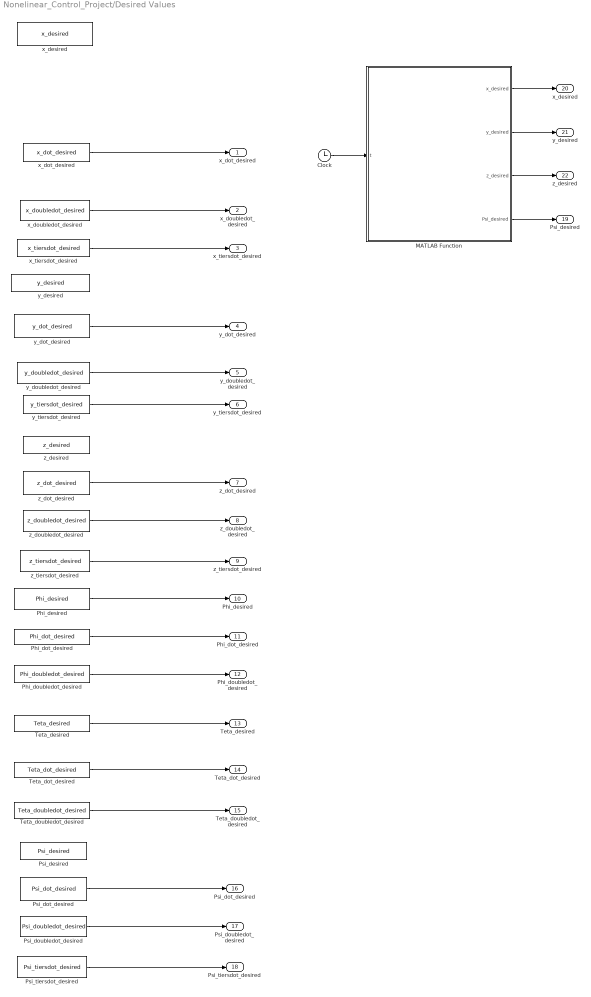
== system Nonelinear_Control_Project/Desired Values  ==
  Clock : Clock
  MATLAB Function : MATLAB Function  TreatAsAtomicUnit=on
  Phi_desired : Constant  Value=Phi_desired
  Phi_dot_desired : Constant  Value=Phi_dot_desired
  Phi_doubledot_desired : Constant  Value=Phi_doubledot_desired
  Psi_desired : Constant  Value=Psi_desired
  Psi_dot_desired : Constant  Value=Psi_dot_desired
  Psi_doubledot_desired : Constant  Value=Psi_doubledot_desired
  Psi_tiersdot_desired : Constant  Value=Psi_tiersdot_desired
  Teta_desired : Constant  Value=Teta_desired
  Teta_dot_desired : Constant  Value=Teta_dot_desired
  Teta_doubledot_desired : Constant  Value=Teta_doubledot_desired
  x_desired : Constant  Value=x_desired
  x_dot_desired : Constant  Value=x_dot_desired
  x_doubledot_desired : Constant  Value=x_doubledot_desired
  x_tiersdot_desired : Constant  Value=x_tiersdot_desired
  y_desired : Constant  Value=y_desired
  y_dot_desired : Constant  Value=y_dot_desired
  y_doubledot_desired : Constant  Value=y_doubledot_desired
  y_tiersdot_desired : Constant  Value=y_tiersdot_desired
  z_desired : Constant  Value=z_desired
  z_dot_desired : Constant  Value=z_dot_desired
  z_doubledot_desired : Constant  Value=z_doubledot_desired
  z_tiersdot_desired : Constant  Value=z_tiersdot_desired
  "x_dot_desired " : Outport
  "x_doubledot_desired " : Outport  Port=2
  "x_tiersdot_desired " : Outport  Port=3
  "y_dot_desired " : Outport  Port=4
  "y_doubledot_desired " : Outport  Port=5
  "y_tiersdot_desired " : Outport  Port=6
  "z_dot_desired " : Outport  Port=7
  "z_doubledot_desired " : Outport  Port=8
  "z_tiersdot_desired " : Outport  Port=9
  "Phi_desired " : Outport  Port=10
  "Phi_dot_desired " : Outport  Port=11
  "Phi_doubledot_desired " : Outport  Port=12
  "Teta_desired " : Outport  Port=13
  "Teta_dot_desired  " : Outport  Port=14
  "Teta_doubledot_desired " : Outport  Port=15
  "Psi_dot_desired " : Outport  Port=16
  "Psi_doubledot_desired " : Outport  Port=17
  "Psi_tiersdot_desired " : Outport  Port=18
  "Psi_desired " : Outport  Port=19
  "x_desired " : Outport  Port=20
  "y_desired " : Outport  Port=21
  "z_desired " : Outport  Port=22
  wires:
  y_dot_desired/1 -> "y_dot_desired "/1
  z_tiersdot_desired/1 -> "z_tiersdot_desired "/1
  x_doubledot_desired/1 -> "x_doubledot_desired "/1
  Teta_dot_desired/1 -> "Teta_dot_desired  "/1
  x_tiersdot_desired/1 -> "x_tiersdot_desired "/1
  z_dot_desired/1 -> "z_dot_desired "/1
  y_doubledot_desired/1 -> "y_doubledot_desired "/1
  Teta_doubledot_desired/1 -> "Teta_doubledot_desired "/1
  z_doubledot_desired/1 -> "z_doubledot_desired "/1
  Teta_desired/1 -> "Teta_desired "/1
  Phi_desired/1 -> "Phi_desired "/1
  y_tiersdot_desired/1 -> "y_tiersdot_desired "/1
  x_dot_desired/1 -> "x_dot_desired "/1
  Phi_doubledot_desired/1 -> "Phi_doubledot_desired "/1
  Phi_dot_desired/1 -> "Phi_dot_desired "/1
  Psi_tiersdot_desired/1 -> "Psi_tiersdot_desired "/1
  Psi_dot_desired/1 -> "Psi_dot_desired "/1
  Psi_doubledot_desired/1 -> "Psi_doubledot_desired "/1
  Clock/1 -> MATLAB Function/1(t)
  MATLAB Function/4(Psi_desired) -> "Psi_desired "/1
  MATLAB Function/1(x_desired) -> "x_desired "/1
  MATLAB Function/2(y_desired) -> "y_desired "/1
  MATLAB Function/3(z_desired) -> "z_desired "/1

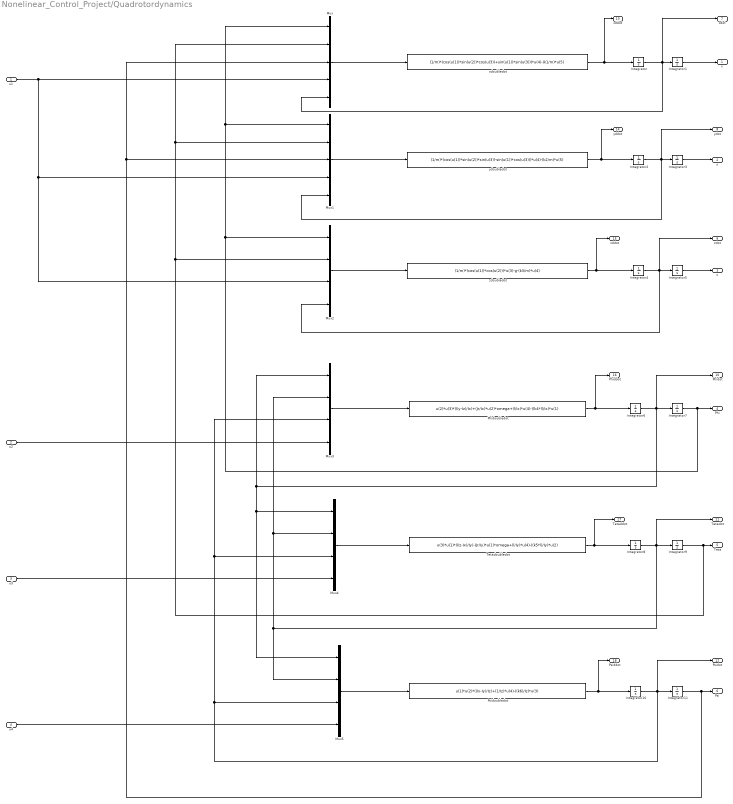
== system Nonelinear_Control_Project/Quadrotordynamics ==
  u1 : Inport
  u2 : Inport  Port=2
  u3 : Inport  Port=3
  u4 : Inport  Port=4
  Integrator{,1..11} (12 alike) : Integrator
  Mux : Mux  Inputs=5
  Mux1 : Mux  Inputs=5
  Mux{2..5} (4 alike) : Mux
  Phidoubledot : Fcn  Expr=u(2)*u(3)*((Iy-Iz)/Ix)+(Jr/Ix)*u(2)*omega+(l/Ix)*u(4)-((k4*l)/Ix)*u(1)
  Psidoubledot : Fcn  Expr=u(1)*u(2)*((Ix-Iy)/Iz)+(1/Iz)*u(4)-((k6)/Iz)*u(3)
  Tetadoubledot : Fcn  Expr=u(3)*u(1)*((Iz-Ix)/Iy)-(Jr/Iy)*u(1)*omega+(l/Iy)*u(4)-((k5*l)/Iy)*u(2)
  xdoubledot : Fcn  Expr=(1/m)*(cos(u(1))*sin(u(2))*cos(u(3))+sin(u(1))*sin(u(3)))*u(4)-(k1/m)*u(5)
  ydoubledot : Fcn  Expr=(1/m)*(cos(u(1))*sin(u(2))*sin(u(3))-sin(u(1))*cos(u(3)))*u(4)-(k2/m)*u(5)
  zdoubledot : Fcn  Expr=(1/m)*(cos(u(1))*cos(u(2)))*u(3)-g-(k3/m)*u(4)
  x : Outport
  y : Outport  Port=2
  z : Outport  Port=3
  Phi : Outport  Port=4
  Teta : Outport  Port=5
  Psi : Outport  Port=6
  xdot : Outport  Port=7
  ydot : Outport  Port=8
  zdot : Outport  Port=9
  Phidot : Outport  Port=10
  Tetadot : Outport  Port=11
  Psidot : Outport  Port=12
  xddot : Outport  Port=13
  yddot : Outport  Port=14
  zddot : Outport  Port=15
  Phiddot : Outport  Port=16
  Tetaddot : Outport  Port=17
  Psiddot : Outport  Port=18
  wires:
  ydoubledot/1 -> yddot/1, Integrator2/1
  Psidoubledot/1 -> Psiddot/1, Integrator10/1
  Integrator10/1 -> Psidot/1, Mux5/3, Mux4/3, Mux3/3, Integrator11/1
  Integrator6/1 -> Phidot/1, Mux5/1, Mux4/1, Mux3/1, Integrator7/1
  Phidoubledot/1 -> Phiddot/1, Integrator6/1
  Tetadoubledot/1 -> Tetaddot/1, Integrator8/1
  Integrator8/1 -> Tetadot/1, Mux5/2, Mux4/2, Mux3/2, Integrator9/1
  Integrator7/1 -> Mux/1, Mux1/1, Mux2/1, Phi/1
  xdoubledot/1 -> xddot/1, Integrator/1
  Integrator2/1 -> Mux1/5, ydot/1, Integrator3/1
  zdoubledot/1 -> zddot/1, Integrator4/1
  Integrator3/1 -> y/1
  Integrator4/1 -> Integrator5/1, zdot/1, Mux2/4
  Integrator/1 -> xdot/1, Mux/5, Integrator1/1
  Integrator9/1 -> Mux2/2, Mux1/2, Mux/2, Teta/1
  Integrator1/1 -> x/1
  Integrator5/1 -> z/1
  Integrator11/1 -> Mux1/3, Mux/3, Psi/1
  Mux/1 -> xdoubledot/1
  Mux1/1 -> ydoubledot/1
  Mux2/1 -> zdoubledot/1
  u1/1 -> Mux/4, Mux1/4, Mux2/3
  u2/1 -> Mux3/4
  u4/1 -> Mux5/4
  u3/1 -> Mux4/4
  Mux3/1 -> Phidoubledot/1
  Mux4/1 -> Tetadoubledot/1
  Mux5/1 -> Psidoubledot/1

== system Nonelinear_Control_Project/Subsystem ==
  u1 : Inport
  Phi : Inport  Port=2
  Psi : Inport  Port=3
  Mux : Mux  Inputs=3
  Mux1 : Mux  Inputs=2
  c1 : Fcn  Expr=(12*m)/(u(1)*cos(u(2))*cos(u(3)))
  c2 : Fcn  Expr=(8*m)/(u(1)*cos(u(2))*cos(u(3)))
  c5 : Fcn  Expr=(-12*m)/(u(1)*cos(u(2)))
  c6 : Fcn  Expr=(-8*m)/(u(1)*cos(u(2)))
  "c1 " : Outport
  "c2 " : Outport  Port=2
  "c5 " : Outport  Port=3
  "c6 " : Outport  Port=4
  wires:
  c5/1 -> "c5 "/1
  c1/1 -> "c1 "/1
  c2/1 -> "c2 "/1
  c6/1 -> "c6 "/1
  u1/1 -> Mux/1, Mux1/1
  Phi/1 -> Mux/2
  Psi/1 -> Mux/3, Mux1/2
  Mux/1 -> c2/1, c1/1
  Mux1/1 -> c5/1, c6/1

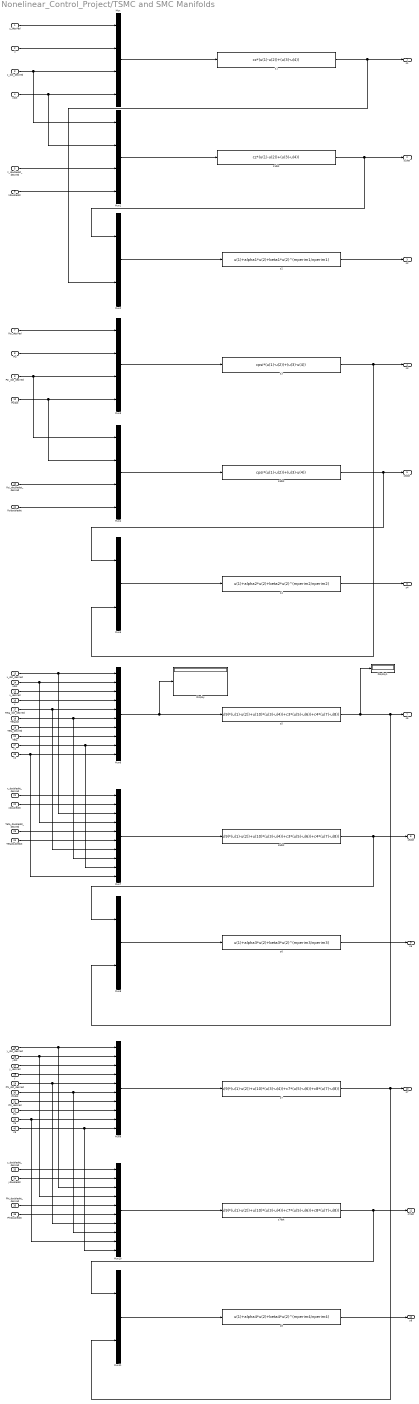
== system Nonelinear_Control_Project/TSMC and SMC Manifolds ==
  "z_desired " : Inport
  z : Inport  Port=2
  z_dot_desired : Inport  Port=3
  "zdot " : Inport  Port=4
  z_doubledot_desired : Inport  Port=5
  zdoubledot : Inport  Port=6
  "Psi_desired " : Inport  Port=7
  Psi : Inport  Port=8
  Psi_dot_desired : Inport  Port=9
  Psidot : Inport  Port=10
  Psidoubledot : Inport  Port=11
  Psi_doubledot_desired : Inport  Port=12
  x_dot_desired : Inport  Port=13
  xdot : Inport  Port=14
  x_desired : Inport  Port=15
  x : Inport  Port=16
  Teta_dot_desired : Inport  Port=17
  Tetadot : Inport  Port=18
  Teta_desired : Inport  Port=19
  Teta : Inport  Port=20
  x_doubledot_desired : Inport  Port=21
  xdoubledot : Inport  Port=22
  Teta_doubledot_desired : Inport  Port=23
  Tetadoubledot : Inport  Port=24
  y_dot_desired : Inport  Port=25
  ydot : Inport  Port=26
  y_desired : Inport  Port=27
  y : Inport  Port=28
  Phi_dot_desired : Inport  Port=29
  Phidot : Inport  Port=30
  Phi_desired : Inport  Port=31
  Phi : Inport  Port=32
  y_doubledot_desired : Inport  Port=33
  ydoubledot : Inport  Port=34
  Phi_doubledot_desired : Inport  Port=35
  Phidoubledot : Inport  Port=36
  c1 : Inport  Port=37
  c2 : Inport  Port=38
  c5 : Inport  Port=39
  c6 : Inport  Port=40
  Display : Display
  Display1 : Display
  Mux{,1,3..4} (4 alike) : Mux
  Mux{6..7,9..10} (4 alike) : Mux  Inputs=10
  Mux{2,5,8,11} (4 alike) : Mux  Inputs=2
  s1 : Fcn  Expr=cz*(u(1)-u(2))+(u(3)-u(4))
  s1dot : Fcn  Expr=cz*(u(1)-u(2))+(u(3)-u(4))
  s2 : Fcn  Expr=u(1)+alpha1*u(2)+beta1*u(2)^(mperim1/nperim1)
  s3 : Fcn  Expr=cpsi*(u(1)-u(2))+(u(3)-u(4))
  s3dot : Fcn  Expr=cpsi*(u(1)-u(2))+(u(3)-u(4))
  s4 : Fcn  Expr=u(1)+alpha2*u(2)+beta2*u(2)^(mperim2/nperim2)
  s5 : Fcn  Expr=u(9)*(u(1)-u(2))+u(10)*(u(3)-u(4))+c3*(u(5)-u(6))+c4*(u(7)-u(8))
  s5dot : Fcn  Expr=u(9)*(u(1)-u(2))+u(10)*(u(3)-u(4))+c3*(u(5)-u(6))+c4*(u(7)-u(8))
  s6 : Fcn  Expr=u(1)+alpha3*u(2)+beta3*u(2)^(mperim3/nperim3)
  s7 : Fcn  Expr=u(9)*(u(1)-u(2))+u(10)*(u(3)-u(4))+c7*(u(5)-u(6))+c8*(u(7)-u(8))
  s7dot : Fcn  Expr=u(9)*(u(1)-u(2))+u(10)*(u(3)-u(4))+c7*(u(5)-u(6))+c8*(u(7)-u(8))
  s8 : Fcn  Expr=u(1)+alpha4*u(2)+beta4*u(2)^(mperim4/nperim4)
  "s1 " : Outport
  "s1dot " : Outport  Port=2
  "s2 " : Outport  Port=3
  "s3 " : Outport  Port=4
  "s3dot " : Outport  Port=5
  "s4 " : Outport  Port=6
  "s5 " : Outport  Port=7
  "s5dot  " : Outport  Port=8
  "s6 " : Outport  Port=9
  "s7 " : Outport  Port=10
  "s7dot " : Outport  Port=11
  "s8 " : Outport  Port=12
  wires:
  Mux/1 -> s1/1
  "z_desired "/1 -> Mux/1
  z/1 -> Mux/2
  z_dot_desired/1 -> Mux/3, Mux1/1
  "zdot "/1 -> Mux/4, Mux1/2
  Mux1/1 -> s1dot/1
  zdoubledot/1 -> Mux1/4
  z_doubledot_desired/1 -> Mux1/3
  Mux2/1 -> s2/1
  s1/1 -> Mux2/2, "s1 "/1
  s1dot/1 -> Mux2/1, "s1dot "/1
  s2/1 -> "s2 "/1
  s3/1 -> Mux5/2, "s3 "/1
  Mux3/1 -> s3/1
  Mux4/1 -> s3dot/1
  s3dot/1 -> Mux5/1, "s3dot "/1
  Psidoubledot/1 -> Mux4/4
  Psi_dot_desired/1 -> Mux4/1, Mux3/3
  Psidot/1 -> Mux4/2, Mux3/4
  Psi/1 -> Mux3/2
  "Psi_desired "/1 -> Mux3/1
  Psi_doubledot_desired/1 -> Mux4/3
  s4/1 -> "s4 "/1
  Mux5/1 -> s4/1
  Mux6/1 -> Display/1, s5/1
  s5/1 -> Display1/1, Mux8/2, "s5 "/1
  x_dot_desired/1 -> Mux6/1, Mux7/3
  xdot/1 -> Mux7/4, Mux6/2
  x_desired/1 -> Mux6/3
  x/1 -> Mux6/4
  Teta_dot_desired/1 -> Mux7/7, Mux6/5
  Tetadot/1 -> Mux7/8, Mux6/6
  Teta_desired/1 -> Mux6/7
  Teta/1 -> Mux6/8
  s5dot/1 -> Mux8/1, "s5dot  "/1
  Mux7/1 -> s5dot/1
  x_doubledot_desired/1 -> Mux7/1
  xdoubledot/1 -> Mux7/2
  Teta_doubledot_desired/1 -> Mux7/5
  Tetadoubledot/1 -> Mux7/6
  s6/1 -> "s6 "/1
  Mux8/1 -> s6/1
  Phidoubledot/1 -> Mux10/6
  y_dot_desired/1 -> Mux9/1, Mux10/3
  ydoubledot/1 -> Mux10/2
  s7/1 -> Mux11/2, "s7 "/1
  Mux9/1 -> s7/1
  s8/1 -> "s8 "/1
  y_desired/1 -> Mux9/3
  Phi_doubledot_desired/1 -> Mux10/5
  y_doubledot_desired/1 -> Mux10/1
  Phi/1 -> Mux9/8
  Phi_desired/1 -> Mux9/7
  Mux10/1 -> s7dot/1
  ydot/1 -> Mux10/4, Mux9/2
  y/1 -> Mux9/4
  Phi_dot_desired/1 -> Mux10/7, Mux9/5
  s7dot/1 -> Mux11/1, "s7dot "/1
  Phidot/1 -> Mux10/8, Mux9/6
  Mux11/1 -> s8/1
  c1/1 -> Mux6/9, Mux7/9
  c2/1 -> Mux6/10, Mux7/10
  c5/1 -> Mux9/9, Mux10/9
  c6/1 -> Mux9/10, Mux10/10

== system Nonelinear_Control_Project/Airplane Dynamics/AnglesBlock ==
  V : Inport
  W : Inport  Port=2
  U : Inport  Port=3
  Atan2 : Trigonometry  Operator=atan2
  Derivative : Derivative
  Derivative1 : Derivative
  Divide : Product  Inputs=*/
  Scope : Scope
  Sin : Trigonometry  Operator=asin
  "beta " : Outport
  alpha : Outport  Port=2
  betadot : Outport  Port=3
  alphadot : Outport  Port=4
  wires:
  U/1 -> Atan2/2, Divide/2
  W/1 -> Atan2/1
  V/1 -> Divide/1
  Atan2/1 -> Derivative1/1, Scope/1, alpha/1
  Sin/1 -> Derivative/1, "beta "/1
  Divide/1 -> Sin/1
  Derivative/1 -> betadot/1
  Derivative1/1 -> alphadot/1

== system Nonelinear_Control_Project/Airplane Dynamics/Angular Velocities (P,Q,R) ==
  LT : Inport
  LAB : Inport  Port=2
  MT : Inport  Port=3
  MAB : Inport  Port=4
  NT : Inport  Port=5
  NAB : Inport  Port=6
  PBlock : Subsystem
  QBlock : Subsystem
  RBlock : Subsystem
  Scope : Scope
  P : Outport
  R : Outport  Port=2
  Q : Outport  Port=3
  wires:
  PBlock/2(Pdot) -> RBlock/3(Pdot)
  PBlock/1(P) -> RBlock/5(P), QBlock/3(P), P/1
  RBlock/2("Rdot ") -> PBlock/3(Rdot)
  LT/1 -> PBlock/2(LT)
  MAB/1 -> QBlock/1(MAB)
  LAB/1 -> PBlock/1(LAB)
  RBlock/1(R) -> R/1, PBlock/4(R), QBlock/4(R)
  NAB/1 -> RBlock/1(NAB)
  NT/1 -> RBlock/2(NT)
  MT/1 -> QBlock/2(MT)
  QBlock/1(Q) -> PBlock/5(Q), RBlock/4(Q), Scope/1, Q/1

== system Nonelinear_Control_Project/Airplane Dynamics/Body Aerodynamic Forces and Moments (FAxB,FAyB,FAzB,LAB,MAB,NAB) ==
  FAxS : Inport
  FAyS : Inport  Port=2
  alpha : Inport  Port=3
  beta : Inport  Port=4
  FAzS : Inport  Port=5
  LAS : Inport  Port=6
  MAS : Inport  Port=7
  NAS : Inport  Port=8
  FAxBBlock : Subsystem
  FAyBBlock : Subsystem
  FAzBBlock : Subsystem
  LABBlock : Subsystem
  MABBlock : Subsystem
  NABBlock : Subsystem
  FAxB : Outport
  FAyB : Outport  Port=2
  FAzB : Outport  Port=3
  LAB : Outport  Port=4
  MAB : Outport  Port=5
  NAB : Outport  Port=6
  wires:
  LAS/1 -> NABBlock/1(LAS), MABBlock/1(LAS), LABBlock/1(LAS)
  NAS/1 -> NABBlock/3(NAS), LABBlock/3(NAS)
  MAS/1 -> NABBlock/2(MAS), LABBlock/2(MAS), MABBlock/2(MAS)
  FAyS/1 -> FAzBBlock/2(FAyS), FAyBBlock/2(FAyS), FAxBBlock/2(FAyS)
  beta/1 -> MABBlock/3(beta), FAxBBlock/5(beta), FAyBBlock/3(beta), FAzBBlock/5(beta), NABBlock/5(beta), LABBlock/5(beta)
  FAzS/1 -> FAxBBlock/3(FAzS), FAzBBlock/3(FAzS)
  MABBlock/1(MAB) -> MAB/1
  FAxS/1 -> FAyBBlock/1(FAxS), FAzBBlock/1(FAxS), FAxBBlock/1(FAxS)
  NABBlock/1(NAB) -> NAB/1
  LABBlock/1(LAB) -> LAB/1
  alpha/1 -> FAzBBlock/4(alpha), FAxBBlock/4(alpha), NABBlock/4(alpha), LABBlock/4(alpha)
  FAxBBlock/1(FAxB) -> FAxB/1
  FAyBBlock/1(FAyB) -> FAyB/1
  FAzBBlock/1(FAzB) -> FAzB/1

== system Nonelinear_Control_Project/Airplane Dynamics/Dynamic Pressure ==
  U : Inport
  V : Inport  Port=2
  W : Inport  Port=3
  Add : Sum  Inputs=+++
  Constant : Constant  Value=2
  Constant1 : Constant  Value=2
  Constant2 : Constant  Value=2
  Divide : Product  Inputs=**/
  Divide1 : Product  Inputs=**/
  Divide2 : Product  Inputs=**/
  Multiply : Product
  Multiply1 : Product
  Multiply2 : Product
  Ro : Constant  Value=Ro
  Ro1 : Constant  Value=Ro
  Ro2 : Constant  Value=Ro
  q1 : Outport
  wires:
  Constant2/1 -> Divide2/3
  Add/1 -> q1/1
  Multiply2/1 -> Divide2/2
  V/1 -> Multiply1/1, Multiply1/2
  Divide2/1 -> Add/3
  Constant/1 -> Divide/3
  Multiply1/1 -> Divide1/2
  Divide1/1 -> Add/2
  U/1 -> Multiply/2, Multiply/1
  Ro2/1 -> Divide2/1
  Multiply/1 -> Divide/2
  W/1 -> Multiply2/1, Multiply2/2
  Divide/1 -> Add/1
  Ro1/1 -> Divide1/1
  Constant1/1 -> Divide1/3
  Ro/1 -> Divide/1

== system Nonelinear_Control_Project/Airplane Dynamics/Euler's Angles (Phi,Theta,Psi) ==
  R : Inport
  Q : Inport  Port=2
  P : Inport  Port=3
  PhiBlock : Subsystem
  PsiBlock : Subsystem
  ThetaBlock : Subsystem
  Psi : Outport
  Phi : Outport  Port=2
  Theta : Outport  Port=3
  wires:
  P/1 -> PhiBlock/1(P)
  ThetaBlock/1(Theta) -> PhiBlock/3(Theta), Theta/1, PsiBlock/3("Theta ")
  PhiBlock/1(Phi) -> PsiBlock/2("Phi "), ThetaBlock/1(Phi), Phi/1
  Q/1 -> PsiBlock/1(Q), ThetaBlock/3(Q), PhiBlock/2(Q)
  R/1 -> PsiBlock/4("R "), ThetaBlock/2(R), PhiBlock/4(R)
  PsiBlock/1(Psi) -> Psi/1

== system Nonelinear_Control_Project/Airplane Dynamics/GBlock ==
  Theta : Inport
  "Phi " : Inport  Port=2
  Cos : Trigonometry  Operator=cos
  Cos1 : Trigonometry  Operator=cos
  Gain : Gain  Gain=-1
  "Gravityl Acceleration " : Constant  Value=g
  Multiply : Product
  Multiply1 : Product  Inputs=3
  Multiply2 : Product  Inputs=3
  Scope : Scope
  Scope1 : Scope
  Scope2 : Scope
  Trigonometric Function : Trigonometry
  Trigonometric Function1 : Trigonometry
  gx : Outport
  gy : Outport  Port=2
  gz : Outport  Port=3
  wires:
  Multiply2/1 -> Scope2/1, gz/1
  "Gravityl Acceleration "/1 -> Multiply1/1, Multiply2/1, Multiply/2
  Theta/1 -> Cos1/1, Trigonometric Function/1
  "Phi "/1 -> Trigonometric Function1/1, Cos/1
  Multiply/1 -> Scope/1, gx/1
  Multiply1/1 -> Scope1/1, gy/1
  Trigonometric Function1/1 -> Multiply1/2
  Cos1/1 -> Multiply2/2, Multiply1/3
  Cos/1 -> Multiply2/3
  Trigonometric Function/1 -> Gain/1
  Gain/1 -> Multiply/1

== system Nonelinear_Control_Project/Airplane Dynamics/Linear Velocities (U,V,W) ==
  FAxB : Inport
  FTx : Inport  Port=2
  FAyB : Inport  Port=3
  FTy : Inport  Port=4
  gx : Inport  Port=5
  gy : Inport  Port=6
  gz : Inport  Port=7
  FAzB : Inport  Port=8
  FTz : Inport  Port=9
  R : Inport  Port=10
  P : Inport  Port=11
  Q : Inport  Port=12
  Add : Sum  Inputs=+-
  Scope : Scope
  Scope2 : Scope
  Scope3 : Scope
  UBlock : Subsystem
  VBlock : Subsystem
  WBlock : Subsystem
  V : Outport
  U : Outport  Port=2
  W : Outport  Port=3
  delU : Outport  Port=4
  wires:
  VBlock/1(V) -> Scope/1, V/1, WBlock/5(V), UBlock/7(V)
  FTx/1 -> UBlock/3("FTx ")
  FAxB/1 -> UBlock/2("FAxB ")
  Q/1 -> UBlock/4("Q "), WBlock/6("Q ")
  R/1 -> UBlock/6("R "), VBlock/5(R)
  FTz/1 -> WBlock/3("FTz ")
  P/1 -> VBlock/6("P "), WBlock/4("P ")
  gy/1 -> VBlock/1(gy)
  FAyB/1 -> VBlock/2("FAyB ")
  gx/1 -> UBlock/1(gx)
  FTy/1 -> VBlock/3("FTy ")
  FAzB/1 -> WBlock/2("FAzB ")
  WBlock/1(W) -> VBlock/7(W), UBlock/5(W), Scope3/1, W/1
  gz/1 -> WBlock/1(gz)
  UBlock/1(U) -> WBlock/7("U "), VBlock/4("U "), Add/2, Add/1, Scope2/1, U/1
  Add/1 -> delU/1

== system Nonelinear_Control_Project/Airplane Dynamics/Navigation ==
  U : Inport
  V : Inport  Port=2
  W : Inport  Port=3
  Phi : Inport  Port=4
  Theta : Inport  Port=5
  Psi : Inport  Port=6
  XInertiaBlock : Subsystem
  YInertiaBlock : Subsystem
  ZInertiaBlock : Subsystem
  XInertia : Outport
  YInertia : Outport  Port=2
  ZInertia : Outport  Port=3
  wires:
  XInertiaBlock/1(XInertia) -> XInertia/1
  Phi/1 -> ZInertiaBlock/4(Phi), YInertiaBlock/4(Phi), XInertiaBlock/4(Phi)
  ZInertiaBlock/1(ZInertia) -> ZInertia/1
  V/1 -> XInertiaBlock/2(V), YInertiaBlock/2(V), ZInertiaBlock/2(V)
  Theta/1 -> ZInertiaBlock/5(Theta), YInertiaBlock/5(Theta), XInertiaBlock/5(Theta)
  U/1 -> ZInertiaBlock/1(U), YInertiaBlock/1(U), XInertiaBlock/1(U)
  Psi/1 -> XInertiaBlock/6(Psi), YInertiaBlock/6(Psi)
  W/1 -> YInertiaBlock/3(W), ZInertiaBlock/3(W), XInertiaBlock/3(W)
  YInertiaBlock/1(YInertia) -> YInertia/1

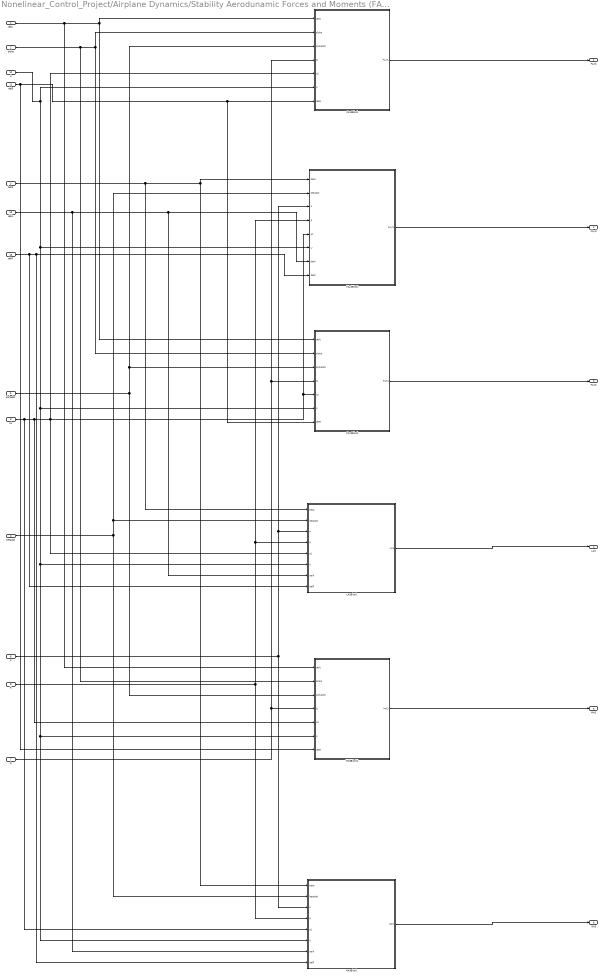
== system Nonelinear_Control_Project/Airplane Dynamics/Stability Aerodunamic Forces and Moments (FAxS,FAyS,FAzS,LAS,MAS,NAS) ==
  delU : Inport
  alpha : Inport  Port=2
  beta : Inport  Port=3
  "betadot " : Inport  Port=4
  alphadot : Inport  Port=5
  P : Inport  Port=6
  Q : Inport  Port=7
  R : Inport  Port=8
  q1 : Inport  Port=9
  delA : Inport  Port=10
  delE : Inport  Port=11
  U : Inport  Port=12
  delR : Inport  Port=13
  FAxSBlock : Subsystem
  FAySBlock : Subsystem
  FAzSBlock : Subsystem
  LASBlock : Subsystem
  MASBlock1 : Subsystem
  NASBlock : Subsystem
  FAxS : Outport
  FAyS : Outport  Port=2
  FAzS : Outport  Port=3
  LAS : Outport  Port=4
  MAS : Outport  Port=5
  NAS : Outport  Port=6
  wires:
  LASBlock/1(LAS) -> LAS/1
  alphadot/1 -> FAxSBlock/3(alphadot), FAzSBlock/3(alphadot), MASBlock1/3(alphadot)
  P/1 -> LASBlock/3(P), FAySBlock/3(P), NASBlock/3(P)
  R/1 -> FAySBlock/4(R), LASBlock/4(R), NASBlock/4(R)
  Q/1 -> MASBlock1/4(Q), FAzSBlock/4(Q), FAxSBlock/4(Q)
  FAzSBlock/1(FAzS) -> FAzS/1
  beta/1 -> LASBlock/1(beta), NASBlock/1(beta), FAySBlock/1(beta)
  "betadot "/1 -> FAySBlock/2(betadot), LASBlock/2(betadot), NASBlock/2(betadot)
  NASBlock/1(NAS) -> NAS/1
  FAySBlock/1(FAyS) -> FAyS/1
  alpha/1 -> MASBlock1/2(alpha), FAzSBlock/2(alpha), FAxSBlock/2(alpha)
  FAxSBlock/1(FAxS) -> FAxS/1
  delU/1 -> MASBlock1/1(delU), FAzSBlock/1(delU), FAxSBlock/1(delU)
  MASBlock1/1(MAS) -> MAS/1
  q1/1 -> NASBlock/5(q1), MASBlock1/5(q1), FAzSBlock/5(q1), FAySBlock/5(q1), LASBlock/5(q1), FAxSBlock/5(q1)
  U/1 -> NASBlock/6(U), MASBlock1/6(U), LASBlock/6(U), FAzSBlock/6(U), FAySBlock/6(U), FAxSBlock/6(U)
  delE/1 -> MASBlock1/7(delE), FAzSBlock/7(delE), FAxSBlock/7(delE)
  delA/1 -> NASBlock/7(delA), LASBlock/7(delA), FAySBlock/7(delA)
  delR/1 -> LASBlock/8(delR), NASBlock/8(delR), FAySBlock/8(delR)
